simulink model "Feedback_Configuration_12"  (R2020a)
settings: Solver=VariableStepAuto  StartTime=0.0  StopTime=75  RelTol=1e-3
libraries: cstblocks x2
settings Model: Creator=geral  LastModifiedBy=geral

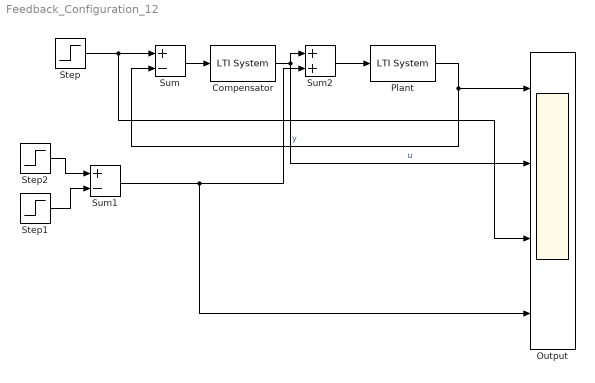
== system Feedback_Configuration_12 ==
  Compensator : cstblocks/LTI System  sys=C  IC=[]
  Output : Scope  NumInputPorts=4
  Plant : cstblocks/LTI System  sys=tf10  IC=[]
  Step : Step  Time=0.1  After=0.7  SampleTime=0
  Step1 : Step  Time=25  After=0.1  SampleTime=0
  Step2 : Step  Time=20  After=0.1  SampleTime=0
  Sum : Sum  Inputs=+-
  Sum1 : Sum  Inputs=+-
  Sum2 : Sum
  wires:
  Sum/1 -> Compensator/1
  Plant/1 -> Sum/2, Output/1  "y"
  Step/1 -> Output/3, Sum/1
  Step2/1 -> Sum1/1
  Step1/1 -> Sum1/2
  Sum2/1 -> Plant/1
  Compensator/1 -> Output/2, Sum2/1  "u"
  Sum1/1 -> Output/4, Sum2/2
